simulink model "fig7_71"  (Simulink 7.9)
settings: Solver=ode45  StartTime=0.0  StopTime=2.0  RelTol=1e-3
settings Model: Creator=abbas  LastModifiedBy=abbas
settings OptimizationCC: InitFltsAndDblsToZero=on
settings DebuggingCC: FcnCallInpInsideContextMsg=Use local settings  StrictBusMsg=Warning
settings GRTTargetCC: CombineOutputUpdateFcns=off  GRTInterface=on

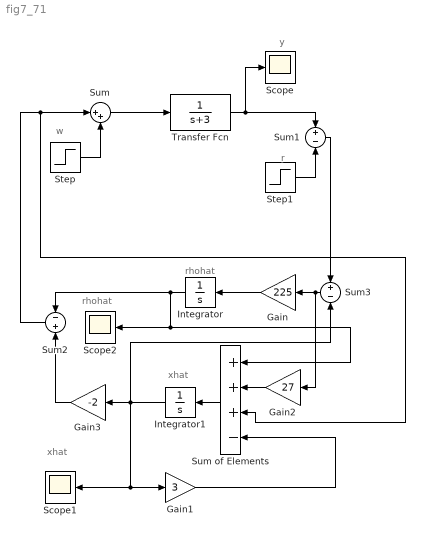
== system fig7_71 ==
  note: w
  note: r
  note: rhohat
  note: xhat
  note: y
  note: rhohat
  note: xhat
  Gain : Gain  Gain=225
  Gain1 : Gain  Gain=3
  Gain2 : Gain  Gain=27
  Gain3 : Gain  Gain=-2
  Integrator : Integrator
  Integrator1 : Integrator
  Scope : Scope
  Scope1 : Scope
  Scope2 : Scope
      settings: SaveName=ScopeData2
  Step : Step  Time=0.5  SampleTime=0
  Step1 : Step  Time=0  SampleTime=0
  Sum : Sum  Inputs=|++
  Sum of Elements : Sum  Inputs=+++-
  Sum1 : Sum  Inputs=+-
  Sum2 : Sum  Inputs=-+
  Sum3 : Sum  Inputs=+-
  Transfer Fcn : TransferFcn  Denominator=[1 3]
  wires:
  Step/1 -> Sum/2
  Step1/1 -> Sum1/2
  Sum2/1 -> Sum/1, Sum of Elements/3
  Sum/1 -> Transfer Fcn/1
  Transfer Fcn/1 -> Sum1/1, Scope/1
  Integrator1/1 -> Sum3/2, Gain1/1, Scope1/1, Gain3/1
  Sum1/1 -> Sum3/1
  Gain/1 -> Integrator/1
  Sum3/1 -> Gain/1, Gain2/1
  Gain1/1 -> Sum of Elements/4
  Integrator/1 -> Sum2/1, Sum of Elements/1, Scope2/1
  Sum of Elements/1 -> Integrator1/1
  Gain2/1 -> Sum of Elements/2
  Gain3/1 -> Sum2/2
